simulink model "state_feedback"  (R2026a)
settings: Solver=VariableStepAuto  StopTime=4  MaxStep=1e-3  RelTol=1e-6
undefined symbols (not defined in the file): A, B, C_theta, C_x, K_2
settings Model: Creator=matte  LastModifiedBy=matte
settings OptimizationCC: BooleanDataType=off
settings DebuggingCC: SaveWithParameterizedLinksMsg=none  SignalResolutionControl=TryResolveAllWithWarning
settings HardwareCC: TargetUnknown=on

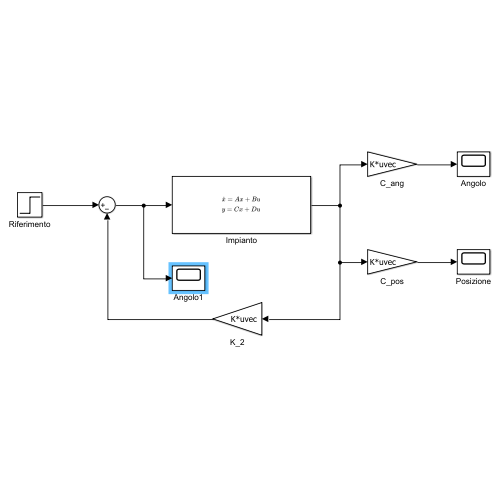
[thumbnail: Simulink's stored preview of the top-level diagram]
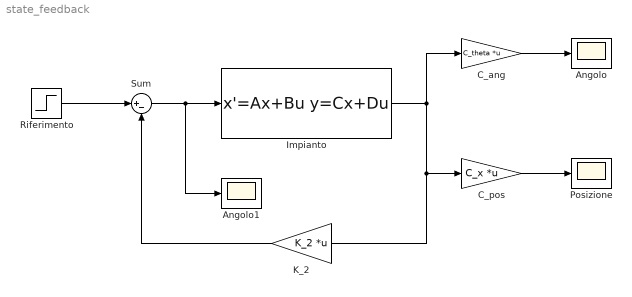
== system state_feedback ==
  Angolo : Scope
      settings: ActiveDisplayYMinimum=-0.023472940601489706  ActiveDisplayYMaximum=0.012215171245289404
  Angolo1 : Scope
      settings: ActiveDisplayYMinimum=-0.53245977644766662  ActiveDisplayYMaximum=1.1702733084941852
  C_ang : Gain  Gain=C_theta  Multiplication=Matrix(K*u) (u vector)
  C_pos : Gain  Gain=C_x  Multiplication=Matrix(K*u) (u vector)
  Impianto : StateSpace  A=A  B=B  C=[1 0 0 0; 0 1 0 0; 0 0 1 0; 0 0 0 1]  D=zeros(4, 1)  InitialCondition=0
  K_2 : Gain  Gain=K_2  Multiplication=Matrix(K*u) (u vector)
  Posizione : Scope
  Riferimento : Step  Time=0
  Sum : Sum  Inputs=|+-
  wires:
  Riferimento/1 -> Sum/1
  Sum/1 -> Angolo1/1, Impianto/1
  Impianto/1 -> K_2/1, C_pos/1, C_ang/1
  C_ang/1 -> Angolo/1
  C_pos/1 -> Posizione/1
  K_2/1 -> Sum/2
